simulink model "pry_grasp_source"  (R2018b)
settings: Solver=FixedStepDiscrete  StartTime=0.0  StopTime=Inf  FixedStep=0.001  RelTol=1e-3
PostLoadFcn:
  | , if any(exist('dsrtsu_mdlpostloadfcn', 'file') ~= 0), dsrtsu_mdlpostloadfcn('Execute', bdroot); end,
undefined symbols (not defined in the file): b, Coulomb_friction, parallel_grasp, q1ini, q2ini, theta1, theta2, theta5, theta6, viscous_friction
libraries: simulink x26
(part 1 of 3)
Description:
  | Standard RTI1007 template.
  | Supported MATLAB version:  R2018b.
settings Model: Tag=RTI1007  DSRTSU_INTERNAL_RTI_VER=530  DSRTSU_INTERNAL_RTI_TYPE=rti1007  RTICANMMDATA=struct('GeneralSetupData',struct('modelroot',['C:\Users\koyama\Documents\MATLAB\zhang\control\pry grasp'],'generalsettings',struct('filesettings',struct('destfolder',struct('Name','RTICANMM_FILES','Check',1),'buildfolder',struct('Name','.','Check',1),'AbsDestfolder',struct('Name',['C:\Users\koyama\Documents\MATLAB\zhang\control\pry grasp\RTICANMM_FILES']),'AbsBuildfolder',struct('Name',['C:\Users\koyama\Documents\MATLAB\zhang\control\pry grasp']))),'options',struct('addpaths',1,'rmpaths',1,'addtrcexclusion',logical(1),'cannavigator',struct('checkmonitoring',0),'show_usrtrc',0,'use_usrtrc',0),'advanced',struct('options',ones(1,100)),'MPSetup',{{}},'RTI',struct('Type','RTI1007','Ver','7.11','Date','02-Nov-2018'),'modelname','pry_grasp','block','pry_grasp'))  DSRTSU_INTERNAL_RTIFPGA=120  Creator=koyama  LastModifiedBy=Zhang Qi
settings OptimizationCC: BlockReduction=off  OptimizeBlockIOStorage=off  BufferReuse=off  GlobalBufferReuse=off  ExpressionFolding=off  LocalBlockOutputs=off  OptimizeDataStoreBuffers=off  BusAssignmentInplaceUpdate=off
settings DebuggingCC: LibraryContextMissingDiagnostic=none
settings HardwareCC: ProdBitPerPointer=32  ProdBitPerSizeT=32  ProdBitPerPtrDiffT=32  ProdLargestAtomicInteger=Integer  ProdEndianess=BigEndian  ProdWordSize=32  ProdHWDeviceType=Custom Processor->Custom  TargetIntDivRoundTo=Zero  TargetEndianess=BigEndian  TargetHWDeviceType=Custom Processor->Custom
settings SFSimCC: SimUseLocalCustomCode=off  MATLABDynamicMemAlloc=off
settings RTWCC: SystemTargetFile=rti1007.tlc  MakeCommand=make_rti  TemplateMakefile=rti1007.tmf  Description=dSPACE DS1007 Hardware Platform  RTWUseLocalCustomCode=off
settings CodeAppCC: StateflowObjectComments=on
settings STFCustomTargetCC: ParMdlRefBuildCompliant=on  SystemTargetFile=rti1007.tlc
settings GRTTargetCC: TargetLangStandard=C89/C90 (ANSI)  CompOptLevelCompliant=off  ConcurrentExecutionCompliant=off  CombineOutputUpdateFcns=off  MatFileLogging=off  CPPClassGenCompliant=off  UseToolchainInfoCompliant=off
settings ConfigComp: CovMetricSettings=dswe

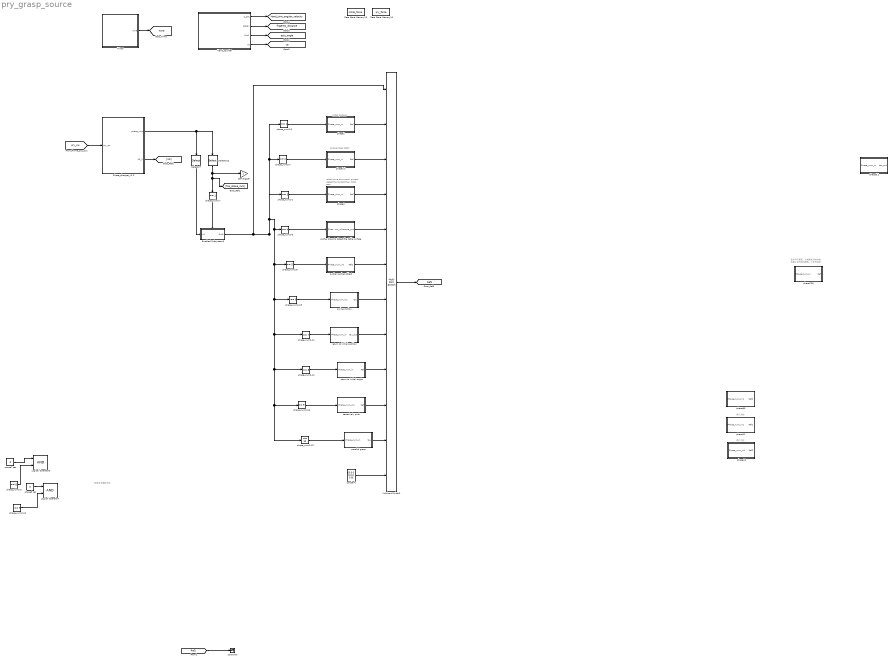
== system pry_grasp_source ==
  note: initial posture
  note: robot move downward,
      | gripper detect the contact
      | then robot stop
  note: gripper keep static
  note: 变为平行抓取，左指两关节向内转，
      | 右指上关节向内旋转，下关节关闭
  note: 所有关节维持不动
  note: 两个力控
  note: 两个力控
  Data Store Memory10 : DataStoreMemory  DataStoreName=pry_force  ReadBeforeWriteMsg=warning  WriteAfterWriteMsg=warning  WriteAfterReadMsg=warning  ShowAdditionalParam=off
  Data Store Memory13 : DataStoreMemory  DataStoreName=initial_force  ReadBeforeWriteMsg=warning  WriteAfterWriteMsg=warning  WriteAfterReadMsg=warning  ShowAdditionalParam=off
  Enabled Subsystem6 : Subsystem  TreatAsAtomicUnit=on
  Hand_counter : Subsystem
  Logical Operator5 : Logic  AllPortsSameDT=off  OutDataTypeStr=boolean
  Logical Operator7 : Logic  AllPortsSameDT=off  OutDataTypeStr=boolean
  Multiport Switch3 : MultiPortSwitch  Inputs=10  DataPortForDefault=Additional data port
  Phase_changer_v2.0 : Subsystem
  Selector12 : Selector  InputPortWidth=2  IndexOptions=Index vector (dialog)  Indices=1  OutputSizes=1
  Selector7 : Selector  InputPortWidth=2  IndexOptions=Index vector (dialog)  Indices=2  OutputSizes=1
  Timer : Subsystem
      mask Display: fprintf('Timer')
  constant : Constant  Value=[0 0 0 0 0 0 0 0]
  controller : Terminator
  parallel grasp : Subsystem
  phase1 : Subsystem
  phase1-1 : Subsystem
  phase10 : Subsystem
  phase11 : Subsystem
  phase2 : Subsystem
  phase6.1 : Subsystem
  phase7 set : Constant  Priority=1  Value=0  OutDataTypeStr=boolean
  phase700 : Subsystem
  phase8 set : Constant  Priority=1  Value=0  OutDataTypeStr=boolean
  phase90 : Subsystem
  phase_num2-1 : simulink/Logic and Bit Operations/Compare To Constant  relop===  const=3  OutDataTypeStr=uint8
  phase_num2-10 : simulink/Logic and Bit Operations/Compare To Constant  relop===  const=9  OutDataTypeStr=uint8
  phase_num2-11 : simulink/Logic and Bit Operations/Compare To Constant  relop===  const=7  OutDataTypeStr=uint8
  phase_num2-12 : simulink/Logic and Bit Operations/Compare To Constant  relop===  const=8  OutDataTypeStr=uint8
  phase_num2-13 : simulink/Logic and Bit Operations/Compare To Constant  relop===  const=10  OutDataTypeStr=uint8
  phase_num2-16 : simulink/Logic and Bit Operations/Compare To Constant  relop===  const=9  OutDataTypeStr=uint8
  phase_num2-19 : simulink/Logic and Bit Operations/Compare To Constant  relop===  const=6  OutDataTypeStr=uint8
  phase_num2-2 : simulink/Logic and Bit Operations/Compare To Constant  relop===  const=8  OutDataTypeStr=uint8
  phase_num2-3 : simulink/Logic and Bit Operations/Compare To Constant  relop===  const=1  OutDataTypeStr=uint8
  phase_num2-5 : simulink/Logic and Bit Operations/Compare To Constant  relop===  const=5  OutDataTypeStr=uint8
  phase_num2-6 : simulink/Logic and Bit Operations/Compare To Constant  relop===  const=4  OutDataTypeStr=uint8
  phase_num2-7 : simulink/Logic and Bit Operations/Compare To Constant  relop===  const=2  OutDataTypeStr=uint8
  phase_num2-x : simulink/Logic and Bit Operations/Compare To Constant  relop===  const=1  OutDataTypeStr=uint8
  prying motion : Subsystem
  pusher drops to detect the table surface : Subsystem
  pusher pushes object : Subsystem
  return to initial angle : Subsystem
  return to initial position : Subsystem
  start trigger : Gain
  tentatively push : Subsystem
  tag scope: Hand_joint_angular_velocity=global, Ref1=global, Time=global, actu_angle=global, fingertip_distance=global, ve=global
  wires:
  Hand_counter/1(q_dot) -> [Hand_joint_angular_velocity]
  Timer/1(time) -> [Time]
  Selector12/1 -> start trigger/1, [Top_phase_num], phase_num2-x/1
  phase_num2-x/1 -> Enabled Subsystem6/Enable
  Selector7/1 -> Enabled Subsystem6/1(In1)
  Multiport Switch3/1 -> [Ref1]
  phase1/1(Ref) -> Multiport Switch3/2
  Phase_changer_v2.0/2(UR_V) -> [UR]
  phase_num2-3/1 -> phase1/1(Phase_num_in)
  phase_num2-1/1 -> phase2/1(Phase_num_in)
  phase_num2-6/1 -> pusher drops to detect the table surface/1(Phase_num_in1)
  phase_num2-5/1 -> pusher pushes object/1(Phase_num_in1)
  phase1-1/1(Ref) -> Multiport Switch3/3
  pusher pushes object/1(Ref2) -> Multiport Switch3/6
  pusher drops to detect the table surface/1(torque_out) -> Multiport Switch3/5
  phase2/1(Ref) -> Multiport Switch3/4
  phase_num2-7/1 -> phase1-1/1(Phase_num_in)
  [pry_sw] -> Phase_changer_v2.0/1(pry_sw)
  Phase_changer_v2.0/1(phase_num) -> Selector7/1, Selector12/1
  [Ref1] -> controller/1
  Enabled Subsystem6/1(Out1) -> phase_num2-3/1, phase_num2-7/1, phase_num2-1/1, phase_num2-19/1, phase_num2-13/1, phase_num2-16/1, phase_num2-12/1, phase_num2-11/1, phase_num2-5/1, phase_num2-6/1, Multiport Switch3/1
  phase_num2-2/1 -> Logical Operator5/2
  phase7 set/1 -> Logical Operator5/1
  phase8 set/1 -> Logical Operator7/1
  phase_num2-10/1 -> Logical Operator7/2
  Hand_counter/2(deltax) -> [fingertip_distance]
  Hand_counter/3(Out1) -> [actu_angle]
  return to initial position/1(tau_out) -> Multiport Switch3/8
  phase_num2-11/1 -> return to initial position/1(Phase_num_in)
  return to initial angle/1(Ref) -> Multiport Switch3/9
  phase_num2-12/1 -> return to initial angle/1(Phase_num_in)
  parallel grasp/1(tau) -> Multiport Switch3/11
  phase_num2-13/1 -> parallel grasp/1(Phase_num_in)
  constant/1 -> Multiport Switch3/12
  tentatively push/1(Ref) -> Multiport Switch3/10
  phase_num2-16/1 -> tentatively push/1(Phase_num_in1)
  Hand_counter/4(ve) -> [ve]
  prying motion/1(tau) -> Multiport Switch3/7
  phase_num2-19/1 -> prying motion/1(Phase_num_in1)

== system pry_grasp_source/Enabled Subsystem6 ==
  In1 : Inport
  Enable : EnablePort
  Out1 : Outport  OutputWhenDisabled=reset  InitialOutput=0
  wires:
  In1/1 -> Out1/1

== system pry_grasp_source/Hand_counter ==
  1/dt : Gain  Gain=1/0.005
  1/dt1 : Gain  Gain=1/0.005
  Delay : Delay  DelayLength=5  InitialCondition=0
  Delay1 : Delay  DelayLength=5  InitialCondition=0
  MATLAB Function : MATLAB Function  TreatAsAtomicUnit=on
  Mux1 : Mux  Inputs=8
  Selector3 : Selector  InputPortWidth=8  IndexOptions=Index vector (dialog)  Indices=1  OutputSizes=1
  Selector4 : Selector  InputPortWidth=8  IndexOptions=Index vector (dialog)  Indices=2  OutputSizes=1
  Selector5 : Selector  InputPortWidth=8  IndexOptions=Index vector (dialog)  Indices=5  OutputSizes=1
  Selector6 : Selector  InputPortWidth=8  IndexOptions=Index vector (dialog)  Indices=6  OutputSizes=1
  Sum : Sum  Inputs=|+-
  Sum1 : Sum  Inputs=|+-
  current angle{1..8} (8 alike) : Constant  Priority=1  Value=0  OutDataTypeStr=boolean
  q_dot : Outport
  deltax : Outport  Port=2
  Out1 : Outport  Port=3
  ve : Outport  Port=4
  wires:
  current angle6/1 -> Mux1/6
  current angle3/1 -> Mux1/3
  current angle7/1 -> Mux1/7
  current angle2/1 -> Mux1/2
  1/dt/1 -> q_dot/1
  current angle4/1 -> Mux1/4
  Sum/1 -> 1/dt/1
  current angle8/1 -> Mux1/8
  Delay/1 -> Sum/2
  current angle5/1 -> Mux1/5
  current angle1/1 -> Mux1/1
  Selector4/1 -> MATLAB Function/2(angle2_deg)
  Selector5/1 -> MATLAB Function/3(angle5_deg)
  Selector6/1 -> MATLAB Function/4(angle6_deg)
  Selector3/1 -> MATLAB Function/1(angle1_deg)
  Mux1/1 -> Delay/1, Sum/1, Out1/1, Selector3/1, Selector4/1, Selector5/1, Selector6/1
  Sum1/1 -> 1/dt1/1
  Delay1/1 -> Sum1/2
  MATLAB Function/1(delta_x) -> deltax/1, Delay1/1, Sum1/1
  1/dt1/1 -> ve/1

== system pry_grasp_source/Phase_changer_v2.0 ==
  pry_sw : Inport
  Data Store Read : DataStoreRead  Priority=3  DataStoreName=phase_num
  Data Store Read4 : DataStoreRead  Priority=3  DataStoreName=UR_V
  Triggered Subsystem : Subsystem  Priority=1  TreatAsAtomicUnit=on
  Triggered Subsystem1 : Subsystem  Priority=2  TreatAsAtomicUnit=on
  phase_num : Outport
  UR_V : Outport  Port=2
  wires:
  Data Store Read/1 -> phase_num/1
  pry_sw/1 -> Triggered Subsystem1/Trigger, Triggered Subsystem/Trigger
  Data Store Read4/1 -> UR_V/1

== system pry_grasp_source/Timer ==
  note: Timer ＆ Eｘ Switch
  Compare To Constant : simulink/Logic and Bit Operations/Compare To Constant  relop=>  const=0  OutDataTypeStr=uint8
  Digital Clock : DigitalClock  SampleTime=0.001
  Logical Operator : Logic  Operator=OR  Inputs=1  AllPortsSameDT=off  OutDataTypeStr=boolean
  Sum2 : Sum  Inputs=|-+
  Switch1 : Switch  Criteria=u2 > Threshold
  Triggered Subsystem : Subsystem  TreatAsAtomicUnit=on
  pry_sw : Constant  Priority=1  Value=0  OutDataTypeStr=boolean
  time : Outport
  tag scope: ex_sw=global, pry_sw=global
  wires:
  Compare To Constant/1 -> Switch1/2, Triggered Subsystem/Trigger
  Digital Clock/1 -> Sum2/2, Switch1/3, Triggered Subsystem/1(In1)
  Triggered Subsystem/1(Out1) -> Switch1/1
  Switch1/1 -> Sum2/1
  Sum2/1 -> time/1  "Enabel_time"
  Logical Operator/1 -> [ex_sw], Compare To Constant/1
  pry_sw/1 -> [pry_sw], Logical Operator/1

== system pry_grasp_source/parallel grasp ==
  Phase_num_in : Inport
  Constant : Constant  Value=parallel_grasp
  tau : Outport
  wires:
  Phase_num_in/1 -> [Phase_Start]
  Constant/1 -> tau/1

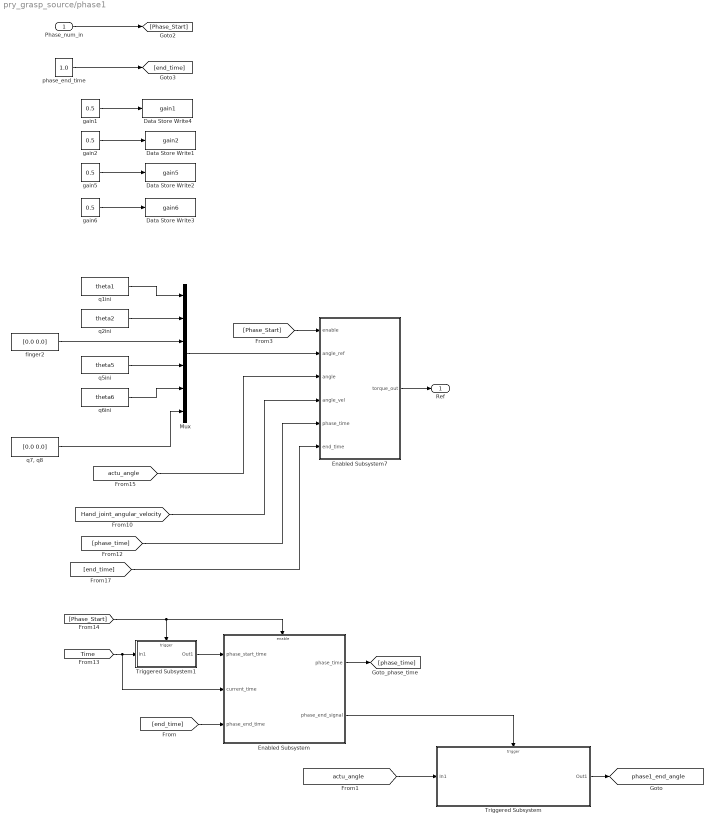
== system pry_grasp_source/phase1 ==
  Phase_num_in : Inport
  Data Store Write1 : DataStoreWrite  DataStoreName=gain2
  Data Store Write2 : DataStoreWrite  DataStoreName=gain5
  Data Store Write3 : DataStoreWrite  DataStoreName=gain6
  Data Store Write4 : DataStoreWrite  DataStoreName=gain1
  Enabled Subsystem : Subsystem  TreatAsAtomicUnit=on
  Enabled Subsystem7 : Subsystem  TreatAsAtomicUnit=on
  Mux : Mux  Inputs=6
  Triggered Subsystem : Subsystem  TreatAsAtomicUnit=on
  Triggered Subsystem1 : Subsystem  TreatAsAtomicUnit=on
  finger2 : Constant  Value=[0.0 0.0]
  gain{1..2,5..6} (4 alike) : Constant  Value=0.5
  phase_end_time : Constant  Value=1.0
  q1ini : Constant  Value=theta1
  q2ini : Constant  Value=theta2
  q5ini : Constant  Value=theta5
  q6ini : Constant  Value=theta6
  "q7, q8" : Constant  Value=[0.0 0.0]
  Ref : Outport
  tag scope: phase1_end_angle=global
  wires:
  Phase_num_in/1 -> [Phase_Start]
  phase_end_time/1 -> [end_time]
  [Hand_joint_angular_velocity] -> Enabled Subsystem7/4(angle_vel)
  [Phase_Start] -> Enabled Subsystem7/1(enable)
  [end_time] -> Enabled Subsystem/3(phase_end_time)
  [Time] -> Triggered Subsystem1/1(In1), Enabled Subsystem/2(current_time)
  Enabled Subsystem/1(phase_time) -> [phase_time]
  [Phase_Start] -> Triggered Subsystem1/Trigger, Enabled Subsystem/Enable
  Enabled Subsystem/2(phase_end_signal) -> Triggered Subsystem/Trigger
  Triggered Subsystem1/1(Out1) -> Enabled Subsystem/1(phase_start_time)
  [actu_angle] -> Enabled Subsystem7/3(angle)
  [phase_time] -> Enabled Subsystem7/5(phase_time)
  [end_time] -> Enabled Subsystem7/6(end_time)
  Enabled Subsystem7/1(torque_out) -> Ref/1
  Mux/1 -> Enabled Subsystem7/2(angle_ref)
  q1ini/1 -> Mux/1
  finger2/1 -> Mux/3
  q5ini/1 -> Mux/4
  "q7, q8"/1 -> Mux/6
  q2ini/1 -> Mux/2
  q6ini/1 -> Mux/5
  gain1/1 -> Data Store Write4/1
  gain2/1 -> Data Store Write1/1
  gain5/1 -> Data Store Write2/1
  gain6/1 -> Data Store Write3/1
  [actu_angle] -> Triggered Subsystem/1(In1)
  Triggered Subsystem/1(Out1) -> [phase1_end_angle]

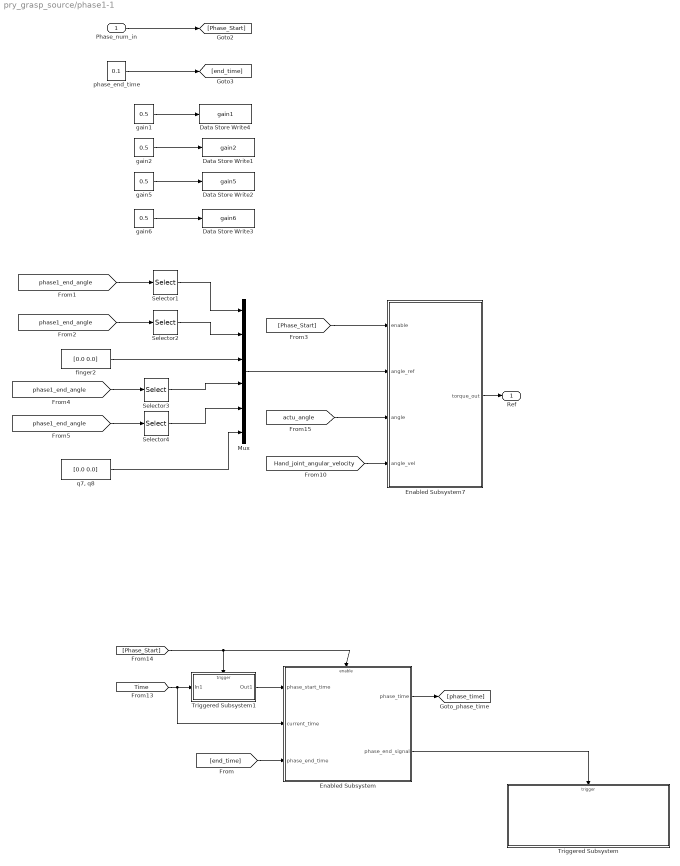
== system pry_grasp_source/phase1-1 ==
  Phase_num_in : Inport
  Data Store Write1 : DataStoreWrite  DataStoreName=gain2
  Data Store Write2 : DataStoreWrite  DataStoreName=gain5
  Data Store Write3 : DataStoreWrite  DataStoreName=gain6
  Data Store Write4 : DataStoreWrite  DataStoreName=gain1
  Enabled Subsystem : Subsystem  TreatAsAtomicUnit=on
  Enabled Subsystem7 : Subsystem  TreatAsAtomicUnit=on
  Mux : Mux  Inputs=6
  Selector1 : Selector  InputPortWidth=8  IndexOptions=Index vector (dialog)  Indices=1  OutputSizes=1
  Selector2 : Selector  InputPortWidth=8  IndexOptions=Index vector (dialog)  Indices=2  OutputSizes=1
  Selector3 : Selector  InputPortWidth=8  IndexOptions=Index vector (dialog)  Indices=5  OutputSizes=1
  Selector4 : Selector  InputPortWidth=8  IndexOptions=Index vector (dialog)  Indices=6  OutputSizes=1
  Triggered Subsystem : Subsystem  TreatAsAtomicUnit=on
  Triggered Subsystem1 : Subsystem  TreatAsAtomicUnit=on
  finger2 : Constant  Value=[0.0 0.0]
  gain{1..2,5..6} (4 alike) : Constant  Value=0.5
  phase_end_time : Constant  Value=0.1
  "q7, q8" : Constant  Value=[0.0 0.0]
  Ref : Outport
  wires:
  Phase_num_in/1 -> [Phase_Start]
  phase_end_time/1 -> [end_time]
  [Hand_joint_angular_velocity] -> Enabled Subsystem7/4(angle_vel)
  [Phase_Start] -> Enabled Subsystem7/1(enable)
  [end_time] -> Enabled Subsystem/3(phase_end_time)
  [Time] -> Triggered Subsystem1/1(In1), Enabled Subsystem/2(current_time)
  Enabled Subsystem/1(phase_time) -> [phase_time]
  [Phase_Start] -> Triggered Subsystem1/Trigger, Enabled Subsystem/Enable
  Enabled Subsystem/2(phase_end_signal) -> Triggered Subsystem/Trigger
  Triggered Subsystem1/1(Out1) -> Enabled Subsystem/1(phase_start_time)
  [actu_angle] -> Enabled Subsystem7/3(angle)
  Enabled Subsystem7/1(torque_out) -> Ref/1
  Mux/1 -> Enabled Subsystem7/2(angle_ref)
  Selector1/1 -> Mux/1
  finger2/1 -> Mux/3
  Selector3/1 -> Mux/4
  "q7, q8"/1 -> Mux/6
  Selector2/1 -> Mux/2
  Selector4/1 -> Mux/5
  gain1/1 -> Data Store Write4/1
  gain2/1 -> Data Store Write1/1
  gain5/1 -> Data Store Write2/1
  gain6/1 -> Data Store Write3/1
  [phase1_end_angle] -> Selector1/1
  [phase1_end_angle] -> Selector2/1
  [phase1_end_angle] -> Selector3/1
  [phase1_end_angle] -> Selector4/1

== system pry_grasp_source/phase10 ==
  note: 给定值
  Phase_num_in1 : Inport
  Data Store Write1 : DataStoreWrite  DataStoreName=gain2
  Data Store Write4 : DataStoreWrite  DataStoreName=gain1
  Enabled Subsystem1 : Subsystem  TreatAsAtomicUnit=on
  Enabled Subsystem3 : Subsystem  TreatAsAtomicUnit=on
  Enabled Subsystem4 : Subsystem  TreatAsAtomicUnit=on
  Selector1 : Selector  InputPortWidth=8  IndexOptions=Index vector (dialog)  Indices=1  OutputSizes=1
  Selector2 : Selector  InputPortWidth=8  IndexOptions=Index vector (dialog)  Indices=2  OutputSizes=1
  Selector3 : Selector  InputPortWidth=8  IndexOptions=Index vector (dialog)  Indices=1  OutputSizes=1
  Selector4 : Selector  InputPortWidth=8  IndexOptions=Index vector (dialog)  Indices=6  OutputSizes=1
  Selector5 : Selector  InputPortWidth=8  IndexOptions=Index vector (dialog)  Indices=5  OutputSizes=1
  Selector6 : Selector  InputPortWidth=8  IndexOptions=Index vector (dialog)  Indices=2  OutputSizes=1
  Selector7 : Selector  InputPortWidth=8  IndexOptions=Index vector (dialog)  Indices=5  OutputSizes=1
  Selector8 : Selector  InputPortWidth=8  IndexOptions=Index vector (dialog)  Indices=6  OutputSizes=1
  Selector9 : Selector  InputPortWidth=8  IndexOptions=Index vector (dialog)  Indices=1  OutputSizes=1
  Triggered Subsystem1 : Subsystem  TreatAsAtomicUnit=on
  Triggered Subsystem4 : Subsystem  TreatAsAtomicUnit=on
  Triggered Subsystem5 : Subsystem  TreatAsAtomicUnit=on
  angle2_the1 : simulink/Logic and Bit Operations/Compare To Constant  relop=>=  const=106  OutDataTypeStr=uint8
  gain1 : Constant
  gain2 : Constant
  phase_end_time1 : Constant  Value=6
  Ref2 : Outport
  wires:
  Triggered Subsystem5/1(Out1) -> Enabled Subsystem3/1(phase_start_time)
  [Time] -> Triggered Subsystem5/1(In1), Enabled Subsystem3/2(current_time)
  Enabled Subsystem3/1(phase_time) -> [phase_time]
  [Phase_Start] -> Triggered Subsystem5/Trigger, Enabled Subsystem3/Enable
  phase_end_time1/1 -> [end_time]
  Phase_num_in1/1 -> [Phase_Start]
  [end_time] -> Enabled Subsystem3/3(phase_end_time)
  Enabled Subsystem3/2(phase_end_signal) -> Triggered Subsystem4/Trigger
  Enabled Subsystem4/1(torque_out) -> Ref2/1
  gain2/1 -> Data Store Write1/1
  gain1/1 -> Data Store Write4/1
  [actu_angle] -> Selector6/1, Selector3/1, Selector5/1, Selector4/1
  [Phase_Start] -> Enabled Subsystem4/1(enable)
  [Hand_joint_angular_velocity] -> Selector7/1, Selector2/1, Selector1/1, Selector8/1
  Selector4/1 -> Enabled Subsystem4/2(angle6)
  Selector5/1 -> Enabled Subsystem4/3(angle5)
  Selector7/1 -> Enabled Subsystem4/4(angular5_vel)
  Selector8/1 -> Enabled Subsystem4/5(angular6_vel)
  Selector3/1 -> Enabled Subsystem4/6(angle1)
  Selector6/1 -> Enabled Subsystem4/7(angle2)
  Selector1/1 -> Enabled Subsystem4/8(angular1_vel)
  Selector2/1 -> Enabled Subsystem4/9(angular2_vel)
  Selector9/1 -> angle2_the1/1
  angle2_the1/1 -> Enabled Subsystem1/1(In1)
  [actu_angle] -> Selector9/1
  [Phase_Start] -> Enabled Subsystem1/Enable
  Enabled Subsystem1/1(Out1) -> Triggered Subsystem1/Trigger
  [fingertip1_vel] -> Enabled Subsystem4/10(vel_x1)

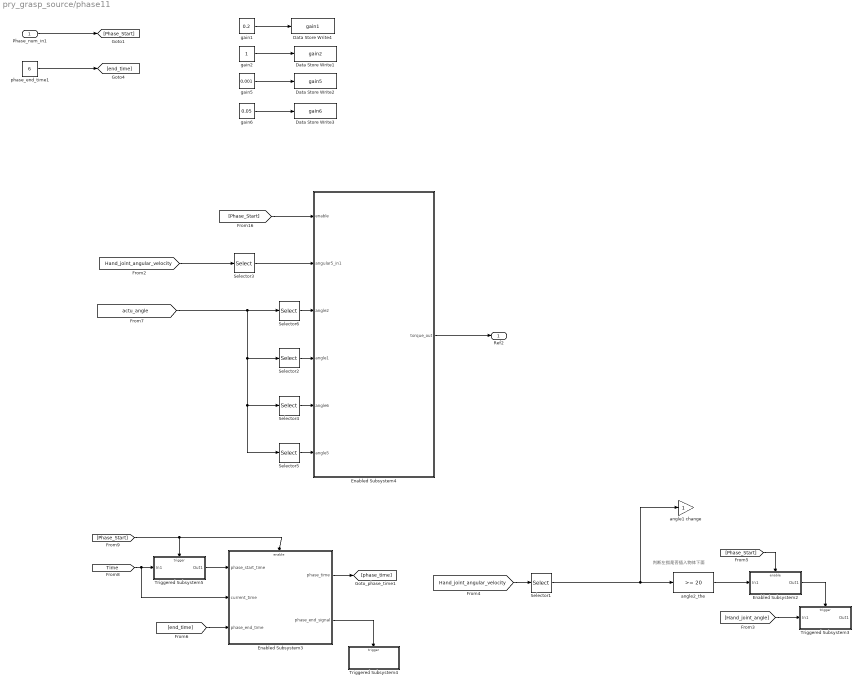
== system pry_grasp_source/phase11 ==
  note: 判断左指是否插入物体下面
  Phase_num_in1 : Inport
  Data Store Write1 : DataStoreWrite  DataStoreName=gain2
  Data Store Write2 : DataStoreWrite  DataStoreName=gain5
  Data Store Write3 : DataStoreWrite  DataStoreName=gain6
  Data Store Write4 : DataStoreWrite  DataStoreName=gain1
  Enabled Subsystem2 : Subsystem  TreatAsAtomicUnit=on
  Enabled Subsystem3 : Subsystem  TreatAsAtomicUnit=on
  Enabled Subsystem4 : Subsystem  TreatAsAtomicUnit=on
  Selector1 : Selector  InputPortWidth=8  IndexOptions=Index vector (dialog)  Indices=1  OutputSizes=1
  Selector2 : Selector  InputPortWidth=8  IndexOptions=Index vector (dialog)  Indices=1  OutputSizes=1
  Selector3 : Selector  InputPortWidth=8  IndexOptions=Index vector (dialog)  Indices=5  OutputSizes=1
  Selector4 : Selector  InputPortWidth=8  IndexOptions=Index vector (dialog)  Indices=6  OutputSizes=1
  Selector5 : Selector  InputPortWidth=8  IndexOptions=Index vector (dialog)  Indices=5  OutputSizes=1
  Selector6 : Selector  InputPortWidth=8  IndexOptions=Index vector (dialog)  Indices=2  OutputSizes=1
  Triggered Subsystem3 : Subsystem  TreatAsAtomicUnit=on
  Triggered Subsystem4 : Subsystem  TreatAsAtomicUnit=on
  Triggered Subsystem5 : Subsystem  TreatAsAtomicUnit=on
  angle1 change : Gain
  angle2_the : simulink/Logic and Bit Operations/Compare To Constant  relop=>=  const=20  OutDataTypeStr=uint8
  gain1 : Constant  Value=0.2
  gain2 : Constant
  gain5 : Constant  Value=0.001
  gain6 : Constant  Value=0.05
  phase_end_time1 : Constant  Value=6
  Ref2 : Outport
  wires:
  Triggered Subsystem5/1(Out1) -> Enabled Subsystem3/1(phase_start_time)
  [Time] -> Triggered Subsystem5/1(In1), Enabled Subsystem3/2(current_time)
  Enabled Subsystem3/1(phase_time) -> [phase_time]
  [Phase_Start] -> Triggered Subsystem5/Trigger, Enabled Subsystem3/Enable
  phase_end_time1/1 -> [end_time]
  Phase_num_in1/1 -> [Phase_Start]
  [end_time] -> Enabled Subsystem3/3(phase_end_time)
  Enabled Subsystem3/2(phase_end_signal) -> Triggered Subsystem4/Trigger
  Enabled Subsystem4/1(torque_out) -> Ref2/1
  gain6/1 -> Data Store Write3/1
  gain2/1 -> Data Store Write1/1
  gain1/1 -> Data Store Write4/1
  gain5/1 -> Data Store Write2/1
  [actu_angle] -> Selector5/1, Selector4/1, Selector2/1, Selector6/1
  Selector6/1 -> Enabled Subsystem4/3(angle2)
  [Phase_Start] -> Enabled Subsystem4/1(enable)
  Selector1/1 -> angle1 change/1, angle2_the/1
  [Phase_Start] -> Enabled Subsystem2/Enable
  [Hand_joint_angle] -> Triggered Subsystem3/1(In1)
  [Hand_joint_angular_velocity] -> Selector1/1
  angle2_the/1 -> Enabled Subsystem2/1(In1)
  Enabled Subsystem2/1(Out1) -> Triggered Subsystem3/Trigger
  [Hand_joint_angular_velocity] -> Selector3/1
  Selector3/1 -> Enabled Subsystem4/2(angular5_in1)
  Selector4/1 -> Enabled Subsystem4/5(angle6)
  Selector5/1 -> Enabled Subsystem4/6(angle5)
  Selector2/1 -> Enabled Subsystem4/4(angle1)

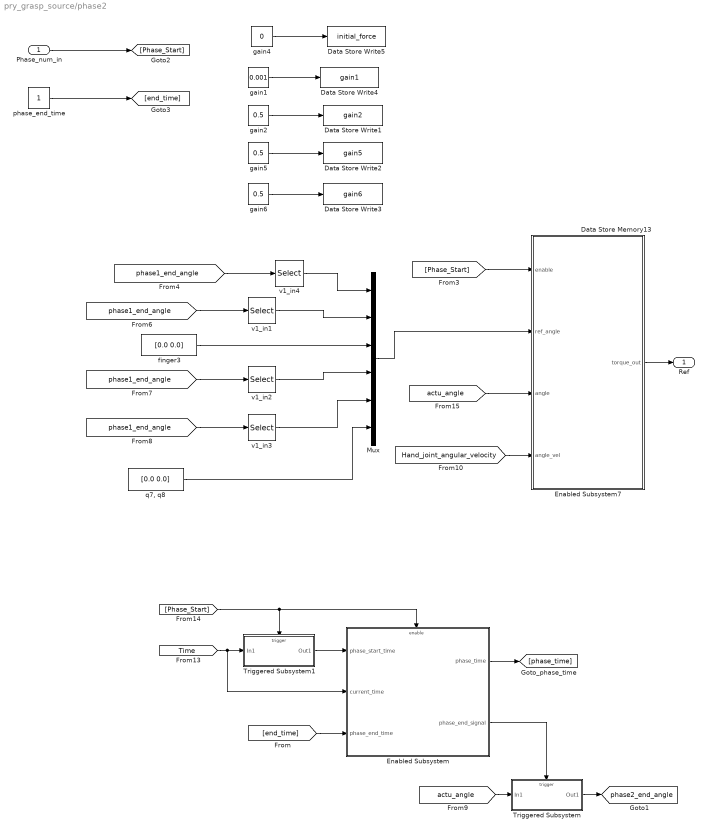
== system pry_grasp_source/phase2 ==
  Phase_num_in : Inport
  Data Store Memory13 : DataStoreMemory  DataStoreName=initial_force  ReadBeforeWriteMsg=warning  WriteAfterWriteMsg=warning  WriteAfterReadMsg=warning  ShowAdditionalParam=off
  Data Store Write1 : DataStoreWrite  DataStoreName=gain2
  Data Store Write2 : DataStoreWrite  DataStoreName=gain5
  Data Store Write3 : DataStoreWrite  DataStoreName=gain6
  Data Store Write4 : DataStoreWrite  DataStoreName=gain1
  Data Store Write5 : DataStoreWrite  DataStoreName=initial_force
  Enabled Subsystem : Subsystem  TreatAsAtomicUnit=on
  Enabled Subsystem7 : Subsystem  TreatAsAtomicUnit=on
  Mux : Mux  Inputs=6
  Triggered Subsystem : Subsystem  TreatAsAtomicUnit=on
  Triggered Subsystem1 : Subsystem  TreatAsAtomicUnit=on
  finger3 : Constant  Value=[0.0 0.0]
  gain1 : Constant  Value=0.001
  gain2 : Constant  Value=0.5
  gain4 : Constant  Value=0
  gain5 : Constant  Value=0.5
  gain6 : Constant  Value=0.5
  phase_end_time : Constant
  "q7, q8" : Constant  Value=[0.0 0.0]
  v1_in1 : Selector  InputPortWidth=8  IndexOptions=Index vector (dialog)  Indices=2  OutputSizes=1
  v1_in2 : Selector  InputPortWidth=8  IndexOptions=Index vector (dialog)  Indices=5  OutputSizes=1
  v1_in3 : Selector  InputPortWidth=8  IndexOptions=Index vector (dialog)  Indices=6  OutputSizes=1
  v1_in4 : Selector  InputPortWidth=8  IndexOptions=Index vector (dialog)  Indices=1  OutputSizes=1
  Ref : Outport
  tag scope: phase2_end_angle=global
  wires:
  Phase_num_in/1 -> [Phase_Start]
  phase_end_time/1 -> [end_time]
  [Hand_joint_angular_velocity] -> Enabled Subsystem7/4(angle_vel)
  [Phase_Start] -> Enabled Subsystem7/1(enable)
  [end_time] -> Enabled Subsystem/3(phase_end_time)
  [Time] -> Triggered Subsystem1/1(In1), Enabled Subsystem/2(current_time)
  Enabled Subsystem/1(phase_time) -> [phase_time]
  [Phase_Start] -> Triggered Subsystem1/Trigger, Enabled Subsystem/Enable
  Enabled Subsystem/2(phase_end_signal) -> Triggered Subsystem/Trigger
  Triggered Subsystem1/1(Out1) -> Enabled Subsystem/1(phase_start_time)
  [actu_angle] -> Enabled Subsystem7/3(angle)
  Enabled Subsystem7/1(torque_out) -> Ref/1
  Mux/1 -> Enabled Subsystem7/2(ref_angle)
  v1_in4/1 -> Mux/1
  finger3/1 -> Mux/3
  v1_in2/1 -> Mux/4
  v1_in1/1 -> Mux/2
  v1_in3/1 -> Mux/5
  "q7, q8"/1 -> Mux/6
  gain2/1 -> Data Store Write1/1
  gain1/1 -> Data Store Write4/1
  gain5/1 -> Data Store Write2/1
  gain6/1 -> Data Store Write3/1
  [phase1_end_angle] -> v1_in4/1
  [phase1_end_angle] -> v1_in1/1
  [phase1_end_angle] -> v1_in2/1
  [phase1_end_angle] -> v1_in3/1
  [actu_angle] -> Triggered Subsystem/1(In1)
  Triggered Subsystem/1(Out1) -> [phase2_end_angle]
  gain4/1 -> Data Store Write5/1

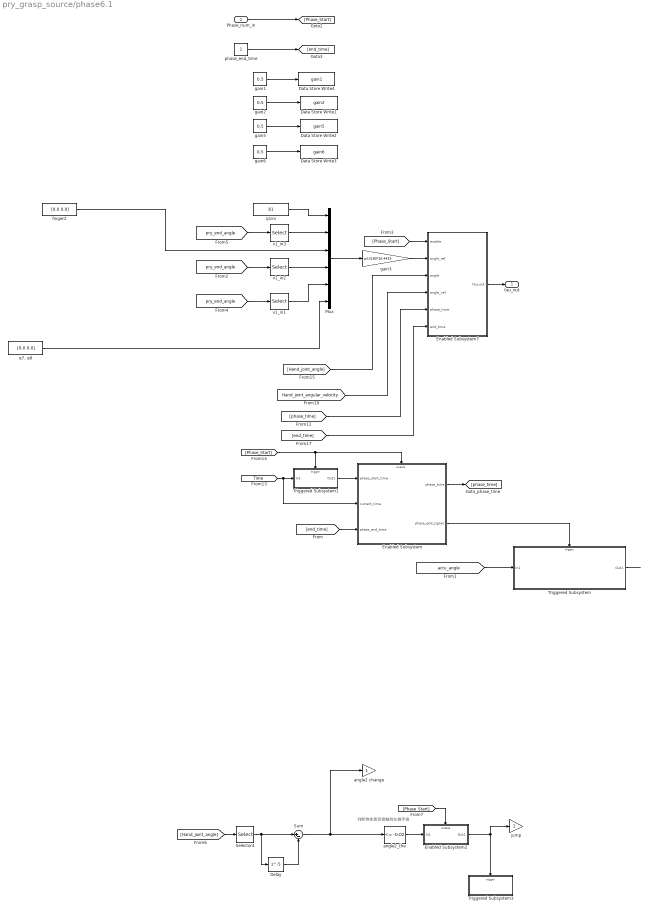
== system pry_grasp_source/phase6.1 ==
  note: 判断物体是否接触到左侧手指
  Phase_num_in : Inport
  Data Store Write1 : DataStoreWrite  DataStoreName=gain2
  Data Store Write2 : DataStoreWrite  DataStoreName=gain5
  Data Store Write3 : DataStoreWrite  DataStoreName=gain6
  Data Store Write4 : DataStoreWrite  DataStoreName=gain1
  Delay : Delay  DelayLength=5  InitialCondition=0
  Enabled Subsystem : Subsystem  TreatAsAtomicUnit=on
  Enabled Subsystem2 : Subsystem  TreatAsAtomicUnit=on
  Enabled Subsystem7 : Subsystem  TreatAsAtomicUnit=on
  Mux : Mux  Inputs=6
  Selector4 : Selector  InputPortWidth=8  IndexOptions=Index vector (dialog)  Indices=2  OutputSizes=1
  Sum : Sum  Inputs=|+-
  Triggered Subsystem : Subsystem  TreatAsAtomicUnit=on
  Triggered Subsystem1 : Subsystem  TreatAsAtomicUnit=on
  Triggered Subsystem3 : Subsystem  TreatAsAtomicUnit=on
  angle2 change : Gain
  angle2_the : simulink/Logic and Bit Operations/Compare To Constant  relop=<=  const=-0.02  OutDataTypeStr=uint8
  finger2 : Constant  Value=[0.0 0.0]
  gain{1..2,5..6} (4 alike) : Constant  Value=0.5
  gain3 : Gain  Gain=pi()/180*16.4423
  jump : Gain
  phase_end_time : Constant
  q1ini : Constant  Value=81
  "q7, q8" : Constant  Value=[0.0 0.0]
  v1_in1 : Selector  InputPortWidth=8  IndexOptions=Index vector (dialog)  Indices=6  OutputSizes=1
  v1_in2 : Selector  InputPortWidth=8  IndexOptions=Index vector (dialog)  Indices=5  OutputSizes=1
  v1_in3 : Selector  InputPortWidth=8  IndexOptions=Index vector (dialog)  Indices=2  OutputSizes=1
  tau_out : Outport
  wires:
  Phase_num_in/1 -> [Phase_Start]
  phase_end_time/1 -> [end_time]
  [Hand_joint_angular_velocity] -> Enabled Subsystem7/4(angle_vel)
  [Phase_Start] -> Enabled Subsystem7/1(enable)
  [end_time] -> Enabled Subsystem/3(phase_end_time)
  [Time] -> Triggered Subsystem1/1(In1), Enabled Subsystem/2(current_time)
  Enabled Subsystem/1(phase_time) -> [phase_time]
  [Phase_Start] -> Triggered Subsystem1/Trigger, Enabled Subsystem/Enable
  Enabled Subsystem/2(phase_end_signal) -> Triggered Subsystem/Trigger
  Triggered Subsystem1/1(Out1) -> Enabled Subsystem/1(phase_start_time)
  [Hand_joint_angle] -> Enabled Subsystem7/3(angle)
  [phase_time] -> Enabled Subsystem7/5(phase_time)
  [end_time] -> Enabled Subsystem7/6(end_time)
  gain3/1 -> Enabled Subsystem7/2(angle_ref)
  Mux/1 -> gain3/1
  q1ini/1 -> Mux/1
  finger2/1 -> Mux/3
  v1_in2/1 -> Mux/4
  "q7, q8"/1 -> Mux/6
  v1_in3/1 -> Mux/2
  v1_in1/1 -> Mux/5
  gain1/1 -> Data Store Write4/1
  gain2/1 -> Data Store Write1/1
  gain5/1 -> Data Store Write2/1
  gain6/1 -> Data Store Write3/1
  [actu_angle] -> Triggered Subsystem/1(In1)
  Triggered Subsystem/1(Out1) -> ?
  [pry_end_angle] -> v1_in2/1
  [pry_end_angle] -> v1_in1/1
  [pry_end_angle] -> v1_in3/1
  Enabled Subsystem7/1(tau_out) -> tau_out/1
  angle2_the/1 -> Enabled Subsystem2/1(In1)
  Sum/1 -> angle2 change/1, angle2_the/1
  [Phase_Start] -> Enabled Subsystem2/Enable
  [Hand_joint_angle] -> Selector4/1
  Selector4/1 -> Delay/1, Sum/1
  Delay/1 -> Sum/2
  Enabled Subsystem2/1(Out1) -> Triggered Subsystem3/Trigger, jump/1

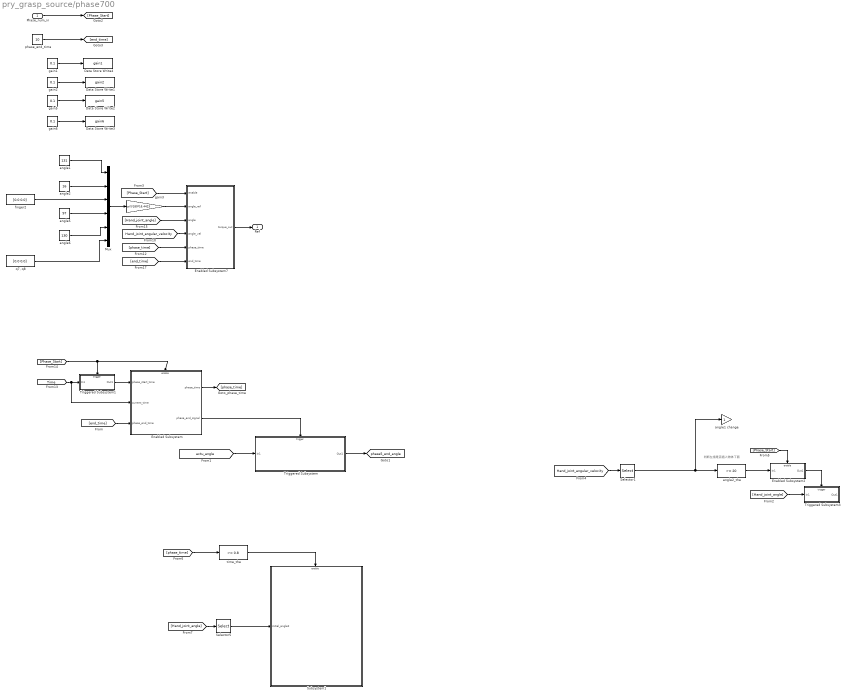
== system pry_grasp_source/phase700 ==
  note: 判断左指是否插入物体下面
  Phase_num_in : Inport
  Data Store Write1 : DataStoreWrite  DataStoreName=gain2
  Data Store Write2 : DataStoreWrite  DataStoreName=gain5
  Data Store Write3 : DataStoreWrite  DataStoreName=gain6
  Data Store Write4 : DataStoreWrite  DataStoreName=gain1
  Enabled Subsystem : Subsystem  TreatAsAtomicUnit=on
  Enabled Subsystem2 : Subsystem  TreatAsAtomicUnit=on
  Enabled Subsystem7 : Subsystem  TreatAsAtomicUnit=on
  Mux : Mux  Inputs=6
  Selector1 : Selector  InputPortWidth=8  IndexOptions=Index vector (dialog)  Indices=1  OutputSizes=1
  Selector5 : Selector  InputPortWidth=8  IndexOptions=Index vector (dialog)  Indices=2  OutputSizes=1
  Subsystem1 : Subsystem
  Triggered Subsystem : Subsystem  TreatAsAtomicUnit=on
  Triggered Subsystem1 : Subsystem  TreatAsAtomicUnit=on
  Triggered Subsystem3 : Subsystem  TreatAsAtomicUnit=on
  angle1 : Constant  Value=131
  angle1 change : Gain
  angle2 : Constant  Value=16
  angle2_the : simulink/Logic and Bit Operations/Compare To Constant  relop=>=  const=20  OutDataTypeStr=uint8
  angle5 : Constant  Value=97
  angle6 : Constant  Value=130
  finger2 : Constant  Value=[0.0 0.0]
  gain{1..2,5..6} (4 alike) : Constant  Value=0.1
  gain3 : Gain  Gain=pi()/180*16.4423
  phase_end_time : Constant  Value=10
  "q7, q8" : Constant  Value=[0.0 0.0]
  time_the : simulink/Logic and Bit Operations/Compare To Constant  relop=>=  const=0.8  OutDataTypeStr=uint8
  Ref : Outport
  tag scope: phase5_end_angle=global
  wires:
  Phase_num_in/1 -> [Phase_Start]
  phase_end_time/1 -> [end_time]
  [end_time] -> Enabled Subsystem/3(phase_end_time)
  [Time] -> Triggered Subsystem1/1(In1), Enabled Subsystem/2(current_time)
  Enabled Subsystem/1(phase_time) -> [phase_time]
  [Phase_Start] -> Triggered Subsystem1/Trigger, Enabled Subsystem/Enable
  Enabled Subsystem/2(phase_end_signal) -> Triggered Subsystem/Trigger
  Triggered Subsystem1/1(Out1) -> Enabled Subsystem/1(phase_start_time)
  Mux/1 -> gain3/1
  finger2/1 -> Mux/3
  "q7, q8"/1 -> Mux/6
  gain1/1 -> Data Store Write4/1
  gain2/1 -> Data Store Write1/1
  gain5/1 -> Data Store Write2/1
  gain6/1 -> Data Store Write3/1
  angle2/1 -> Mux/2
  angle1/1 -> Mux/1
  angle5/1 -> Mux/4
  angle6/1 -> Mux/5
  Enabled Subsystem7/1(torque_out) -> Ref/1
  [end_time] -> Enabled Subsystem7/6(end_time)
  [Hand_joint_angle] -> Enabled Subsystem7/3(angle)
  gain3/1 -> Enabled Subsystem7/2(angle_ref)
  [Hand_joint_angular_velocity] -> Enabled Subsystem7/4(angle_vel)
  [phase_time] -> Enabled Subsystem7/5(phase_time)
  [Phase_Start] -> Enabled Subsystem7/1(enable)
  [actu_angle] -> Triggered Subsystem/1(In1)
  Triggered Subsystem/1(Out1) -> [phase5_end_angle]
  Selector1/1 -> angle1 change/1, angle2_the/1
  Enabled Subsystem2/1(Out1) -> Triggered Subsystem3/Trigger
  [Hand_joint_angular_velocity] -> Selector1/1
  [Phase_Start] -> Enabled Subsystem2/Enable
  [Hand_joint_angle] -> Triggered Subsystem3/1(In1)
  angle2_the/1 -> Enabled Subsystem2/1(In1)
  time_the/1 -> Subsystem1/Enable
  [phase_time] -> time_the/1
  [Hand_joint_angle] -> Selector5/1
  Selector5/1 -> Subsystem1/1(initial_angle2)

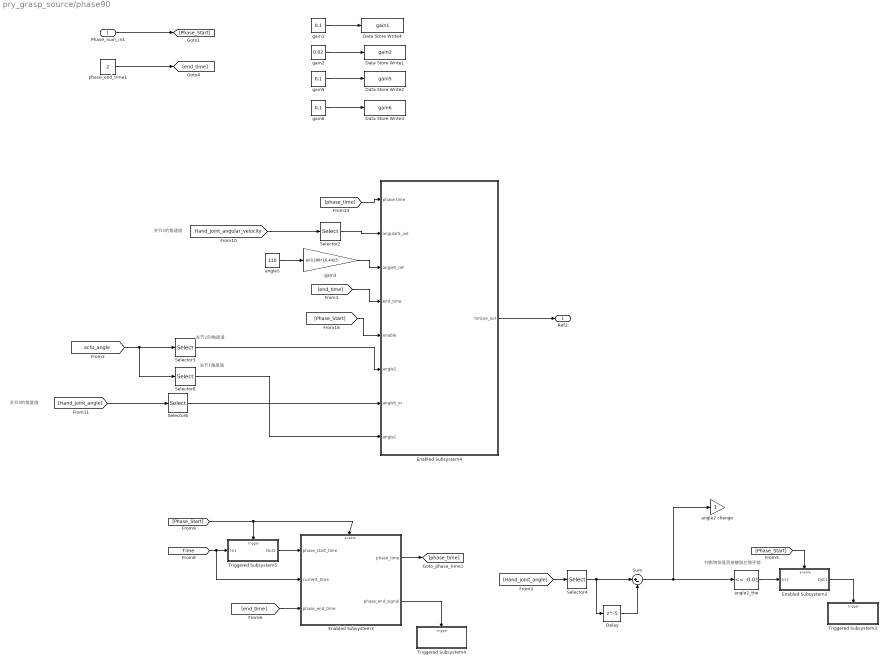
== system pry_grasp_source/phase90 ==
  note: 关节2的角度值
  note: 关节5的角度值
  note: 关节1角度值
  note: 关节5的角速度
  note: 判断物体是否接触到左侧手指
  Phase_num_in1 : Inport
  Data Store Write1 : DataStoreWrite  DataStoreName=gain2
  Data Store Write2 : DataStoreWrite  DataStoreName=gain5
  Data Store Write3 : DataStoreWrite  DataStoreName=gain6
  Data Store Write4 : DataStoreWrite  DataStoreName=gain1
  Delay : Delay  DelayLength=5  InitialCondition=0
  Enabled Subsystem2 : Subsystem  TreatAsAtomicUnit=on
  Enabled Subsystem3 : Subsystem  TreatAsAtomicUnit=on
  Enabled Subsystem4 : Subsystem  TreatAsAtomicUnit=on
  Selector2 : Selector  InputPortWidth=8  IndexOptions=Index vector (dialog)  Indices=5  OutputSizes=1
  Selector3 : Selector  InputPortWidth=8  IndexOptions=Index vector (dialog)  Indices=2  OutputSizes=1
  Selector4 : Selector  InputPortWidth=8  IndexOptions=Index vector (dialog)  Indices=2  OutputSizes=1
  Selector6 : Selector  InputPortWidth=8  IndexOptions=Index vector (dialog)  Indices=5  OutputSizes=1
  Selector8 : Selector  InputPortWidth=8  IndexOptions=Index vector (dialog)  Indices=1  OutputSizes=1
  Sum : Sum  Inputs=|+-
  Triggered Subsystem3 : Subsystem  TreatAsAtomicUnit=on
  Triggered Subsystem4 : Subsystem  TreatAsAtomicUnit=on
  Triggered Subsystem5 : Subsystem  TreatAsAtomicUnit=on
  angle2 change : Gain
  angle2_the : simulink/Logic and Bit Operations/Compare To Constant  relop=<=  const=-0.01  OutDataTypeStr=uint8
  angle5 : Constant  Value=110
  gain1 : Constant  Value=0.1
  gain2 : Constant  Value=0.02
  gain3 : Gain  Gain=pi()/180*16.4423
  gain5 : Constant  Value=0.1
  gain6 : Constant  Value=0.1
  phase_end_time1 : Constant  Value=2
  Ref2 : Outport
  wires:
  Triggered Subsystem5/1(Out1) -> Enabled Subsystem3/1(phase_start_time)
  [Time] -> Triggered Subsystem5/1(In1), Enabled Subsystem3/2(current_time)
  Enabled Subsystem3/1(phase_time) -> [phase_time]
  [Phase_Start] -> Triggered Subsystem5/Trigger, Enabled Subsystem3/Enable
  phase_end_time1/1 -> [end_time]
  Phase_num_in1/1 -> [Phase_Start]
  [end_time] -> Enabled Subsystem3/3(phase_end_time)
  Enabled Subsystem3/2(phase_end_signal) -> Triggered Subsystem4/Trigger
  Enabled Subsystem4/1(torque_out) -> Ref2/1
  Selector3/1 -> Enabled Subsystem4/6(angle2)
  gain6/1 -> Data Store Write3/1
  gain2/1 -> Data Store Write1/1
  gain1/1 -> Data Store Write4/1
  gain5/1 -> Data Store Write2/1
  [Hand_joint_angle] -> Selector6/1
  Selector6/1 -> Enabled Subsystem4/7(angle5_in)
  [Phase_Start] -> Enabled Subsystem4/5(enable)
  [actu_angle] -> Selector8/1, Selector3/1
  Selector8/1 -> Enabled Subsystem4/8(angle1)
  [end_time] -> Enabled Subsystem4/4(end_time)
  angle5/1 -> gain3/1
  gain3/1 -> Enabled Subsystem4/3(angle5_ref)
  [Hand_joint_angular_velocity] -> Selector2/1
  Selector2/1 -> Enabled Subsystem4/2(angular5_vel)
  [phase_time] -> Enabled Subsystem4/1(phase time)
  angle2_the/1 -> Enabled Subsystem2/1(In1)
  Sum/1 -> angle2 change/1, angle2_the/1
  Selector4/1 -> Delay/1, Sum/1
  Delay/1 -> Sum/2
  [Phase_Start] -> Enabled Subsystem2/Enable
  [Hand_joint_angle] -> Selector4/1
  Enabled Subsystem2/1(Out1) -> Triggered Subsystem3/Trigger

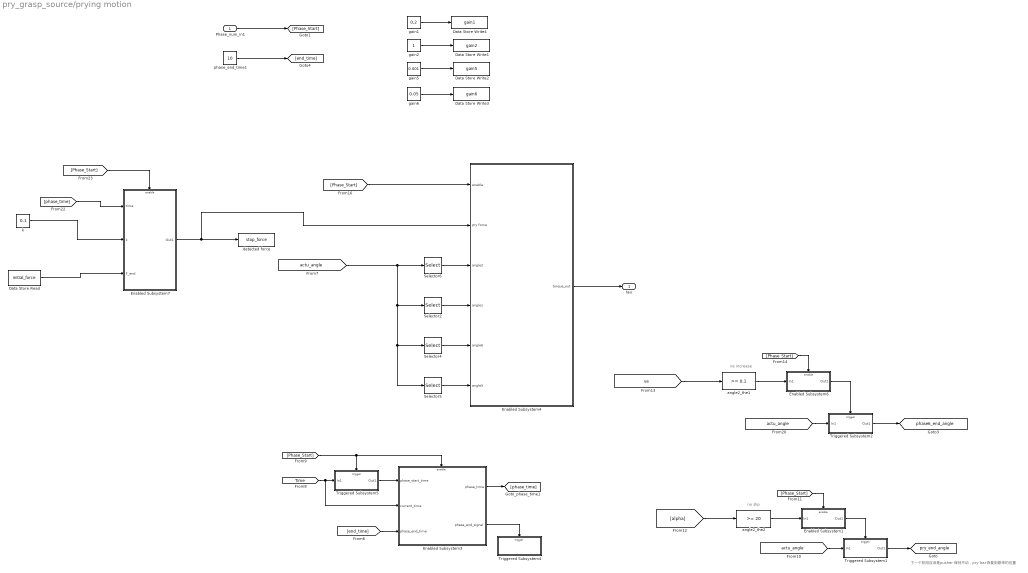
== system pry_grasp_source/prying motion ==
  note: 下一个阶段应该是pusher 保持不动，pry bar 恢复到原来的位置
  note: no slip
  note: ve increase
  Phase_num_in1 : Inport
  Data Store Read : DataStoreRead  DataStoreName=initial_force
  Data Store Write1 : DataStoreWrite  DataStoreName=gain2
  Data Store Write2 : DataStoreWrite  DataStoreName=gain5
  Data Store Write3 : DataStoreWrite  DataStoreName=gain6
  Data Store Write4 : DataStoreWrite  DataStoreName=gain1
  Enabled Subsystem1 : Subsystem  TreatAsAtomicUnit=on
  Enabled Subsystem3 : Subsystem  TreatAsAtomicUnit=on
  Enabled Subsystem4 : Subsystem  TreatAsAtomicUnit=on
  Enabled Subsystem6 : Subsystem  TreatAsAtomicUnit=on
  Enabled Subsystem7 : Subsystem  TreatAsAtomicUnit=on
  Selector2 : Selector  InputPortWidth=8  IndexOptions=Index vector (dialog)  Indices=1  OutputSizes=1
  Selector4 : Selector  InputPortWidth=8  IndexOptions=Index vector (dialog)  Indices=6  OutputSizes=1
  Selector5 : Selector  InputPortWidth=8  IndexOptions=Index vector (dialog)  Indices=5  OutputSizes=1
  Selector6 : Selector  InputPortWidth=8  IndexOptions=Index vector (dialog)  Indices=2  OutputSizes=1
  Triggered Subsystem1 : Subsystem  TreatAsAtomicUnit=on
  Triggered Subsystem2 : Subsystem  TreatAsAtomicUnit=on
  Triggered Subsystem4 : Subsystem  TreatAsAtomicUnit=on
  Triggered Subsystem5 : Subsystem  TreatAsAtomicUnit=on
  angle2_the1 : simulink/Logic and Bit Operations/Compare To Constant  relop=>=  const=0.1  OutDataTypeStr=uint8
  angle2_the2 : simulink/Logic and Bit Operations/Compare To Constant  relop=>=  const=20  OutDataTypeStr=uint8
  detected force : DataStoreWrite  DataStoreName=stop_force
  gain1 : Constant  Value=0.2
  gain2 : Constant
  gain5 : Constant  Value=0.001
  gain6 : Constant  Value=0.05
  k : Constant  Value=0.1
  phase_end_time1 : Constant  Value=10
  tau : Outport
  tag scope: phase6_end_angle=global, pry_end_angle=global
  wires:
  Triggered Subsystem5/1(Out1) -> Enabled Subsystem3/1(phase_start_time)
  [Time] -> Triggered Subsystem5/1(In1), Enabled Subsystem3/2(current_time)
  Enabled Subsystem3/1(phase_time) -> [phase_time]
  [Phase_Start] -> Triggered Subsystem5/Trigger, Enabled Subsystem3/Enable
  phase_end_time1/1 -> [end_time]
  Phase_num_in1/1 -> [Phase_Start]
  [end_time] -> Enabled Subsystem3/3(phase_end_time)
  Enabled Subsystem3/2(phase_end_signal) -> Triggered Subsystem4/Trigger
  Enabled Subsystem4/1(torque_out) -> tau/1
  gain6/1 -> Data Store Write3/1
  gain2/1 -> Data Store Write1/1
  gain1/1 -> Data Store Write4/1
  gain5/1 -> Data Store Write2/1
  [actu_angle] -> Selector5/1, Selector4/1, Selector2/1, Selector6/1
  Selector6/1 -> Enabled Subsystem4/3(angle2)
  [Phase_Start] -> Enabled Subsystem4/1(enable)
  Selector4/1 -> Enabled Subsystem4/5(angle6)
  Selector5/1 -> Enabled Subsystem4/6(angle5)
  Selector2/1 -> Enabled Subsystem4/4(angle1)
  [Phase_Start] -> Enabled Subsystem6/Enable
  [Phase_Start] -> Enabled Subsystem7/Enable
  [ve] -> angle2_the1/1
  [phase_time] -> Enabled Subsystem7/1(time)
  Triggered Subsystem2/1(Out1) -> [phase6_end_angle]
  [actu_angle] -> Triggered Subsystem2/1(In1)
  angle2_the2/1 -> Enabled Subsystem1/1(In1)
  Enabled Subsystem6/1(Out1) -> Triggered Subsystem2/Trigger
  [actu_angle] -> Triggered Subsystem1/1(In1)
  Enabled Subsystem1/1(Out1) -> Triggered Subsystem1/Trigger
  Triggered Subsystem1/1(Out1) -> [pry_end_angle]
  angle2_the1/1 -> Enabled Subsystem6/1(In1)
  k/1 -> Enabled Subsystem7/2(k)
  [Phase_Start] -> Enabled Subsystem1/Enable
  [alpha] -> angle2_the2/1
  Enabled Subsystem7/1(Out1) -> Enabled Subsystem4/2(pry force), detected force/1
  Data Store Read/1 -> Enabled Subsystem7/3(F_end)

== system pry_grasp_source/pusher drops to detect the table surface ==
  Phase_num_in1 : Inport
  Data Store Write1 : DataStoreWrite  DataStoreName=gain2
  Data Store Write2 : DataStoreWrite  DataStoreName=gain5
  Data Store Write3 : DataStoreWrite  DataStoreName=gain6
  Data Store Write4 : DataStoreWrite  DataStoreName=gain1
  Enabled Subsystem3 : Subsystem  TreatAsAtomicUnit=on
  Triggered Subsystem4 : Subsystem  TreatAsAtomicUnit=on
  Triggered Subsystem5 : Subsystem  TreatAsAtomicUnit=on
  friction_compensation model : Subsystem
  gain1 : Constant  Value=0.5
  gain2 : Constant  Value=0.5
  gain5 : Constant  Value=0.5
  gain6 : Constant  Value=2
  phase_end_time1 : Constant  Value=0.1
  torque : Constant  Value=[0 0 0 0 0 0 0 0]
  torque_out : Outport  OutputWhenDisabled=reset  InitialOutput=[0 0 0 0 0 0 0 0]
  tag scope: pusher_angle=global
  wires:
  Triggered Subsystem5/1(Out1) -> Enabled Subsystem3/1(phase_start_time)
  [Time] -> Triggered Subsystem5/1(In1), Enabled Subsystem3/2(current_time)
  Enabled Subsystem3/1(phase_time) -> [phase_time]
  [Phase_Start] -> Triggered Subsystem5/Trigger, Enabled Subsystem3/Enable
  phase_end_time1/1 -> [end_time]
  Phase_num_in1/1 -> [Phase_Start]
  [end_time] -> Enabled Subsystem3/3(phase_end_time)
  Enabled Subsystem3/2(phase_end_signal) -> Triggered Subsystem4/Trigger
  gain6/1 -> Data Store Write3/1
  gain2/1 -> Data Store Write1/1
  gain1/1 -> Data Store Write4/1
  gain5/1 -> Data Store Write2/1
  [actu_angle] -> friction_compensation model/2(angle)
  [Phase_Start] -> friction_compensation model/Enable
  [Hand_joint_angular_velocity] -> friction_compensation model/1(vel)
  friction_compensation model/1(tau_Ref) -> torque_out/1
  torque/1 -> friction_compensation model/4(torque)
  [actu_angle] -> Triggered Subsystem4/1(In1)
  Triggered Subsystem4/1(angle_end) -> [pusher_angle]
  [phase2_end_angle] -> friction_compensation model/3(phase2 end angle)

== system pry_grasp_source/pusher pushes object ==
  Phase_num_in1 : Inport
  Data Store Write1 : DataStoreWrite  DataStoreName=gain2
  Data Store Write2 : DataStoreWrite  DataStoreName=pry_force
  Data Store Write3 : DataStoreWrite  DataStoreName=gain6
  Data Store Write4 : DataStoreWrite  DataStoreName=gain1
  Enabled Subsystem3 : Subsystem  TreatAsAtomicUnit=on
  Enabled Subsystem4 : Subsystem  TreatAsAtomicUnit=on
  Selector1 : Selector  InputPortWidth=8  IndexOptions=Index vector (dialog)  Indices=2  OutputSizes=1
  Selector6 : Selector  InputPortWidth=8  IndexOptions=Index vector (dialog)  Indices=2  OutputSizes=1
  Subsystem1 : Subsystem
  Triggered Subsystem4 : Subsystem  TreatAsAtomicUnit=on
  Triggered Subsystem5 : Subsystem  TreatAsAtomicUnit=on
  gain1 : Constant  Value=0.005
  gain2 : Constant  Value=0.02
  gain5 : Constant  Value=0.15
  gain6 : Constant  Value=0.1
  phase_end_time1 : Constant  Value=3
  Ref2 : Outport
  wires:
  Triggered Subsystem5/1(Out1) -> Enabled Subsystem3/1(phase_start_time)
  [Time] -> Triggered Subsystem5/1(In1), Enabled Subsystem3/2(current_time)
  Enabled Subsystem3/1(phase_time) -> [phase_time]
  [Phase_Start] -> Triggered Subsystem5/Trigger, Enabled Subsystem3/Enable
  phase_end_time1/1 -> [end_time]
  Phase_num_in1/1 -> [Phase_Start]
  [end_time] -> Enabled Subsystem3/3(phase_end_time)
  Enabled Subsystem3/2(phase_end_signal) -> Triggered Subsystem4/Trigger
  Enabled Subsystem4/1(torque) -> Ref2/1
  [actu_angle] -> Selector6/1
  gain2/1 -> Data Store Write1/1
  gain1/1 -> Data Store Write4/1
  [phase_time] -> Enabled Subsystem4/1(phase time)
  gain5/1 -> Data Store Write2/1
  gain6/1 -> Data Store Write3/1
  [ve] -> Subsystem1/1(ve)
  [phase_time] -> Subsystem1/Enable
  Selector6/1 -> Enabled Subsystem4/2("angle2 ")
  [actu_angle] -> Selector1/1
  Selector1/1 -> Enabled Subsystem4/3(angle1)

== system pry_grasp_source/return to initial angle ==
  Phase_num_in : Inport
  Data Store Write1 : DataStoreWrite  DataStoreName=gain2
  Data Store Write2 : DataStoreWrite  DataStoreName=gain5
  Data Store Write3 : DataStoreWrite  DataStoreName=gain6
  Data Store Write4 : DataStoreWrite  DataStoreName=gain1
  Enabled Subsystem : Subsystem  TreatAsAtomicUnit=on
  Enabled Subsystem7 : Subsystem  TreatAsAtomicUnit=on
  Triggered Subsystem : Subsystem  TreatAsAtomicUnit=on
  Triggered Subsystem1 : Subsystem  TreatAsAtomicUnit=on
  gain{1..2,5..6} (4 alike) : Constant  Value=0.5
  phase_end_time : Constant
  q2ini : Constant  Value=q2ini
  Ref : Outport
  wires:
  Phase_num_in/1 -> [Phase_Start]
  phase_end_time/1 -> [end_time]
  [Hand_joint_angular_velocity] -> Enabled Subsystem7/4(angle_vel)
  [Phase_Start] -> Enabled Subsystem7/1(enable)
  [end_time] -> Enabled Subsystem/3(phase_end_time)
  [Time] -> Triggered Subsystem1/1(In1), Enabled Subsystem/2(current_time)
  Enabled Subsystem/1(phase_time) -> [phase_time]
  [Phase_Start] -> Triggered Subsystem1/Trigger, Enabled Subsystem/Enable
  Enabled Subsystem/2(phase_end_signal) -> Triggered Subsystem/Trigger
  Triggered Subsystem1/1(Out1) -> Enabled Subsystem/1(phase_start_time)
  [actu_angle] -> Enabled Subsystem7/3(angle)
  [phase_time] -> Enabled Subsystem7/5(phase_time)
  [end_time] -> Enabled Subsystem7/6(end_time)
  Enabled Subsystem7/1(torque_out) -> Ref/1
  q2ini/1 -> Enabled Subsystem7/2(angle_ref)
  gain1/1 -> Data Store Write4/1
  gain2/1 -> Data Store Write1/1
  gain5/1 -> Data Store Write2/1
  gain6/1 -> Data Store Write3/1

== system pry_grasp_source/return to initial position ==
  Phase_num_in : Inport
  Data Store Write1 : DataStoreWrite  DataStoreName=gain2
  Data Store Write2 : DataStoreWrite  DataStoreName=gain5
  Data Store Write3 : DataStoreWrite  DataStoreName=gain6
  Data Store Write4 : DataStoreWrite  DataStoreName=gain1
  Enabled Subsystem : Subsystem  TreatAsAtomicUnit=on
  Enabled Subsystem7 : Subsystem  TreatAsAtomicUnit=on
  Triggered Subsystem : Subsystem  TreatAsAtomicUnit=on
  Triggered Subsystem1 : Subsystem  TreatAsAtomicUnit=on
  gain{1..2,5..6} (4 alike) : Constant  Value=0.5
  phase_end_time : Constant
  q1ini : Constant  Value=q1ini
  tau_out : Outport
  tag scope: phase6_5_end_angle=global
  wires:
  Phase_num_in/1 -> [Phase_Start]
  phase_end_time/1 -> [end_time]
  [Hand_joint_angular_velocity] -> Enabled Subsystem7/4(angle_vel)
  [Phase_Start] -> Enabled Subsystem7/1(enable)
  [end_time] -> Enabled Subsystem/3(phase_end_time)
  [Time] -> Triggered Subsystem1/1(In1), Enabled Subsystem/2(current_time)
  Enabled Subsystem/1(phase_time) -> [phase_time]
  [Phase_Start] -> Triggered Subsystem1/Trigger, Enabled Subsystem/Enable
  Enabled Subsystem/2(phase_end_signal) -> Triggered Subsystem/Trigger
  Triggered Subsystem1/1(Out1) -> Enabled Subsystem/1(phase_start_time)
  [actu_angle] -> Enabled Subsystem7/3(angle)
  [phase_time] -> Enabled Subsystem7/5(phase_time)
  [end_time] -> Enabled Subsystem7/6(end_time)
  q1ini/1 -> Enabled Subsystem7/2(angle_ref)
  gain1/1 -> Data Store Write4/1
  gain2/1 -> Data Store Write1/1
  gain5/1 -> Data Store Write2/1
  gain6/1 -> Data Store Write3/1
  [actu_angle] -> Triggered Subsystem/1(In1)
  Triggered Subsystem/1(Out1) -> [phase6_5_end_angle]
  Enabled Subsystem7/1(tau_out) -> tau_out/1

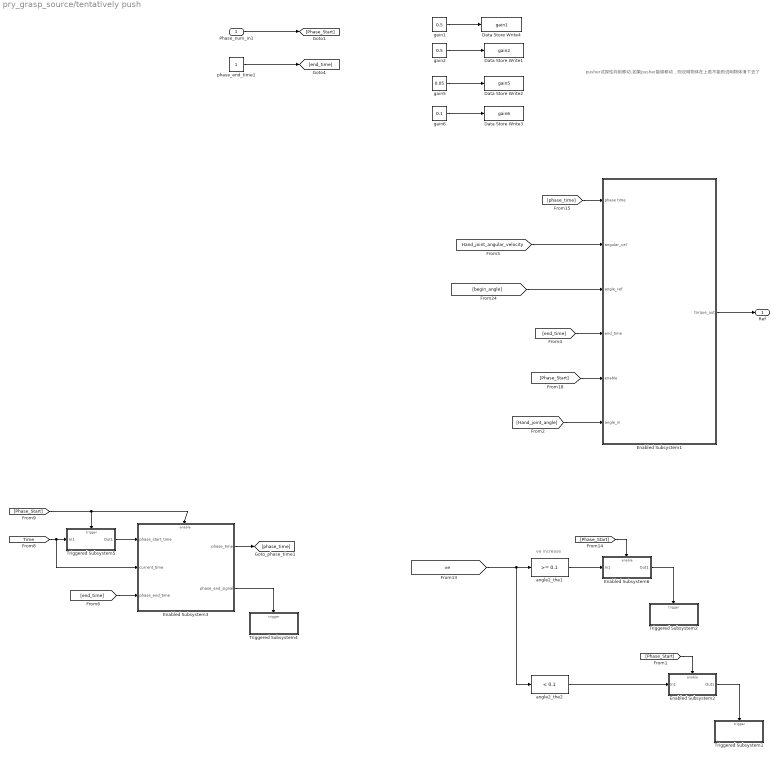
== system pry_grasp_source/tentatively push ==
  note: pusher试探性向前移动,如果pusher能够移动，则说明物体在上若不能则说明物体滑下去了
  note: ve increase
  Phase_num_in1 : Inport
  Data Store Write1 : DataStoreWrite  DataStoreName=gain2
  Data Store Write2 : DataStoreWrite  DataStoreName=gain5
  Data Store Write3 : DataStoreWrite  DataStoreName=gain6
  Data Store Write4 : DataStoreWrite  DataStoreName=gain1
  Enabled Subsystem1 : Subsystem  TreatAsAtomicUnit=on
  Enabled Subsystem2 : Subsystem  TreatAsAtomicUnit=on
  Enabled Subsystem3 : Subsystem  TreatAsAtomicUnit=on
  Enabled Subsystem6 : Subsystem  TreatAsAtomicUnit=on
  Triggered Subsystem1 : Subsystem  TreatAsAtomicUnit=on
  Triggered Subsystem2 : Subsystem  TreatAsAtomicUnit=on
  Triggered Subsystem4 : Subsystem  TreatAsAtomicUnit=on
  Triggered Subsystem5 : Subsystem  TreatAsAtomicUnit=on
  angle2_the1 : simulink/Logic and Bit Operations/Compare To Constant  relop=>=  const=0.1  OutDataTypeStr=uint8
  angle2_the2 : simulink/Logic and Bit Operations/Compare To Constant  relop=<  const=0.1  OutDataTypeStr=uint8
  gain1 : Constant  Value=0.5
  gain2 : Constant  Value=0.5
  gain5 : Constant  Value=0.05
  gain6 : Constant  Value=0.1
  phase_end_time1 : Constant
  Ref : Outport
  wires:
  [Phase_Start] -> Enabled Subsystem1/5(enable)
  [begin_angle] -> Enabled Subsystem1/3(angle_ref)
  [Hand_joint_angular_velocity] -> Enabled Subsystem1/2(angular_vel)
  [end_time] -> Enabled Subsystem1/4(end_time)
  Enabled Subsystem3/2(phase_end_signal) -> Triggered Subsystem4/Trigger
  [Phase_Start] -> Triggered Subsystem5/Trigger, Enabled Subsystem3/Enable
  [Hand_joint_angle] -> Enabled Subsystem1/6(angle_in)
  gain6/1 -> Data Store Write3/1
  Enabled Subsystem1/1(torque_out) -> Ref/1
  gain5/1 -> Data Store Write2/1
  gain1/1 -> Data Store Write4/1
  [end_time] -> Enabled Subsystem3/3(phase_end_time)
  phase_end_time1/1 -> [end_time]
  [phase_time] -> Enabled Subsystem1/1(phase time)
  Triggered Subsystem5/1(Out1) -> Enabled Subsystem3/1(phase_start_time)
  Enabled Subsystem3/1(phase_time) -> [phase_time]
  gain2/1 -> Data Store Write1/1
  Phase_num_in1/1 -> [Phase_Start]
  [Time] -> Triggered Subsystem5/1(In1), Enabled Subsystem3/2(current_time)
  Enabled Subsystem6/1(Out1) -> Triggered Subsystem2/Trigger
  [ve] -> angle2_the2/1, angle2_the1/1
  angle2_the1/1 -> Enabled Subsystem6/1(In1)
  [Phase_Start] -> Enabled Subsystem6/Enable
  angle2_the2/1 -> Enabled Subsystem2/1(In1)
  Enabled Subsystem2/1(Out1) -> Triggered Subsystem1/Trigger
  [Phase_Start] -> Enabled Subsystem2/Enable

== system pry_grasp_source/Phase_changer_v2.0/Triggered Subsystem ==
  Trigger : TriggerPort  VariantControl=(inherit)
  Data Store Write : DataStoreWrite  DataStoreName=phase_num
  initial_phase_num : Constant  Value=[1 1]
  wires:
  initial_phase_num/1 -> Data Store Write/1

== system pry_grasp_source/Phase_changer_v2.0/Triggered Subsystem1 ==
  Trigger : TriggerPort  TriggerType=falling  VariantControl=(inherit)
  Data Store Write : DataStoreWrite  DataStoreName=phase_num
  Data Store Write1 : DataStoreWrite  DataStoreName=i
  Data Store Write2 : DataStoreWrite  DataStoreName=rot_num
  Data Store Write3 : DataStoreWrite  DataStoreName=static_flag
  Data Store Write6 : DataStoreWrite  DataStoreName=UR_V
  i_reset : Constant  Value=0
  initial_UR_V : Constant  Value=0
  initial_phase_num : Constant  Value=[0 0]
  initial_rot_num : Constant  Value=0
  initial_rot_num1 : Constant
  wires:
  initial_phase_num/1 -> Data Store Write/1
  i_reset/1 -> Data Store Write1/1
  initial_rot_num/1 -> Data Store Write2/1
  initial_rot_num1/1 -> Data Store Write3/1
  initial_UR_V/1 -> Data Store Write6/1

== system pry_grasp_source/Timer/Triggered Subsystem ==
  In1 : Inport
  Trigger : TriggerPort  VariantControl=(inherit)
  Out1 : Outport
  wires:
  In1/1 -> Out1/1

== system pry_grasp_source/phase1/Enabled Subsystem ==
  phase_start_time : Inport
  current_time : Inport  Port=2
  phase_end_time : Inport  Port=3
  Enable : EnablePort
  Relational Operator : RelationalOperator  OutDataTypeStr=boolean  RndMeth=Nearest
  Sum : Sum  Inputs=|-+
  phase_time : Outport  OutputWhenDisabled=reset  InitialOutput=0
  phase_end_signal : Outport  Port=2  OutputWhenDisabled=reset  InitialOutput=0
  wires:
  phase_start_time/1 -> Sum/1
  current_time/1 -> Sum/2
  Sum/1 -> phase_time/1, Relational Operator/1
  Relational Operator/1 -> phase_end_signal/1
  phase_end_time/1 -> Relational Operator/2
